simulink model "cheetahSim4trajOpt"  (R2020b)
settings: Solver=ode45  StartTime=0.0  StopTime=simTime  FixedStep=0.001  RelTol=1e-3
values from neighbouring files (symbols this model uses):
  Cd = 1.2    [cheetahTrajOpt.m]    (also in initSim.m; initSim4trajOpt.m)
  p_s = [0; 0; 0]    [cheetahEOM.m]    (also in initSim.m = [0; 0; h_b/2]; initSim4trajOpt.m = [0; 0; h_b/2])
  p_tb = p_b_com__b + [-l_b/2; 0; 0]    [cheetahEOM.m]    (also in initSim.m; initSim4trajOpt.m)
  p_tt_t = [-l_t; 0; 0]    [initSim.m]    (also in initSim4trajOpt.m)
  tau_max = 30    [cheetahTrajOpt.m]    (also in initSim4trajOpt.m)
  v = [v_x; v_y; v_z]    [cheetahEOM.m]    (also in cheetahTrajOpt.m = [10; 2; 0]; initSim.m = 0; initSim4trajOpt.m = [10; 2; 0])
  vert_b = [vert_b; vert_b - [l_b, 0, 0]]    [initSim.m]    (also in initSim4trajOpt.m)
libraries: simulink x2
settings Model: Creator=ricky  LastModifiedBy=ricky
settings SFSimCC: CustomCodeUndefinedFunction=UseInterfaceOnly

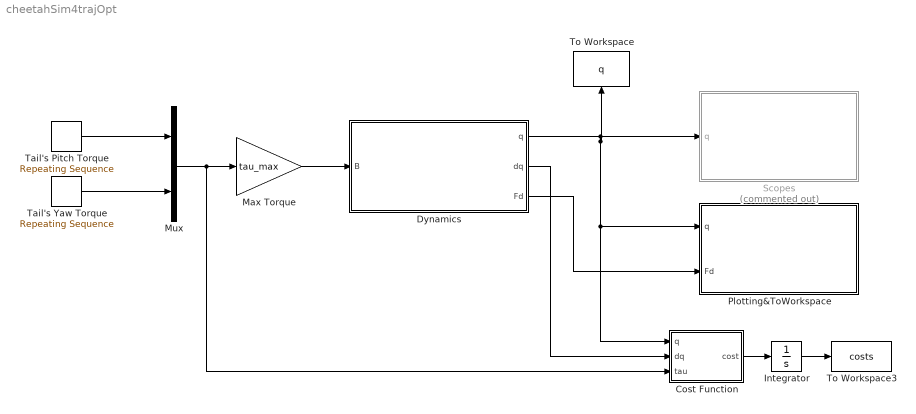
== system cheetahSim4trajOpt ==
  Cost Function : MATLAB Function  TreatAsAtomicUnit=on
  Dynamics : Subsystem
  Integrator : Integrator
  Max Torque : Gain  Gain=tau_max
  Mux : Mux  Inputs=2
  Plotting&ToWorkspace : Subsystem
  Scopes : Subsystem  Commented=on
  Tail's Pitch Torque : simulink/Sources/Repeating Sequence  rep_seq_t=timeVec  rep_seq_y=tau_th
  Tail's Yaw Torque : simulink/Sources/Repeating Sequence  rep_seq_t=timeVec  rep_seq_y=tau_psi
  To Workspace : ToWorkspace  VariableName=q  SampleTime=0.001
  To Workspace3 : ToWorkspace  VariableName=costs  SampleTime=0.001
  wires:
  Dynamics/1(q) -> Cost Function/1(q), Plotting&ToWorkspace/1(q), To Workspace/1, Scopes/1(q)
  Tail's Pitch Torque/1 -> Mux/1
  Tail's Yaw Torque/1 -> Mux/2
  Mux/1 -> Cost Function/3(tau), Max Torque/1
  Max Torque/1 -> Dynamics/1(B)
  Cost Function/1(cost) -> Integrator/1
  Integrator/1 -> To Workspace3/1
  Dynamics/3(Fd) -> Plotting&ToWorkspace/2(Fd)
  Dynamics/2(dq) -> Cost Function/2(dq)

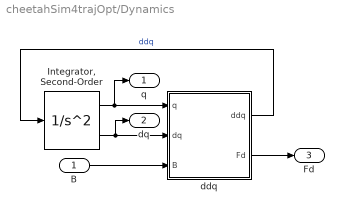
== system cheetahSim4trajOpt/Dynamics ==
  B : Inport
  "Integrator, Second-Order" : SecondOrderIntegrator  ICX=q0  ICDXDT=dq0
  ddq : MATLAB Function  TreatAsAtomicUnit=on
  q : Outport
  dq : Outport  Port=2
  Fd : Outport  Port=3
  wires:
  ddq/1(ddq) -> "Integrator, Second-Order"/1  "ddq"
  "Integrator, Second-Order"/2 -> dq/1, ddq/2(dq)
  "Integrator, Second-Order"/1 -> ddq/1(q), q/1
  B/1 -> ddq/3(B)
  ddq/2(Fd) -> Fd/1

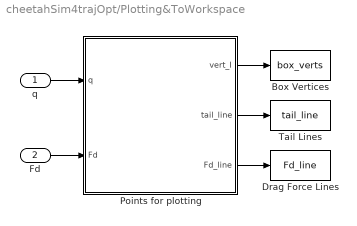
== system cheetahSim4trajOpt/Plotting&ToWorkspace ==
  q : Inport
  Fd : Inport  Port=2
  Box Vertices : ToWorkspace  VariableName=box_verts  SampleTime=-1
  Drag Force Lines : ToWorkspace  VariableName=Fd_line  SampleTime=-1
  Points for plotting : MATLAB Function  TreatAsAtomicUnit=on
  "Tail Lines " : ToWorkspace  VariableName=tail_line  SampleTime=-1
  wires:
  Fd/1 -> Points for plotting/2(Fd)
  Points for plotting/1(vert_I) -> Box Vertices/1
  Points for plotting/2(tail_line) -> "Tail Lines "/1
  q/1 -> Points for plotting/1(q)
  Points for plotting/3(Fd_line) -> Drag Force Lines/1

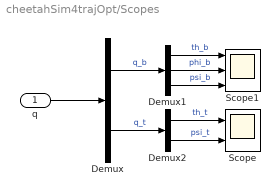
== system cheetahSim4trajOpt/Scopes ==
  q : Inport
  Demux : Demux  Outputs=2
  Demux1 : Demux  Outputs=3
  Demux2 : Demux  Outputs=2
  Scope : Scope  NumInputPorts=2
  Scope1 : Scope  NumInputPorts=3
  wires:
  Demux1/1 -> Scope1/1  "th_b"
  Demux/1 -> Demux1/1  "q_b"
  Demux2/1 -> Scope/1  "th_t"
  q/1 -> Demux/1
  Demux2/2 -> Scope/2  "psi_t"
  Demux1/2 -> Scope1/2  "phi_b"
  Demux1/3 -> Scope1/3  "psi_b"
  Demux/2 -> Demux2/1  "q_t"

== matlab function cheetahSim4trajOpt/Cost Function ==
  data: q input; dq input; tau input; cost output
function cost = cost(q, dq, tau)
    q_b = q(2:3);
    dq_b = dq(2:3);
    
    alpha = 0.5;
    cost = alpha*(q_b'*q_b + dq_b'*dq_b) + (1-alpha)*tau'*tau;
end

== matlab function cheetahSim4trajOpt/Plotting&ToWorkspace/Points for plotting ==
  data: q input; Fd input; vert_I output; tail_line output; p_s parameter; vert_b parameter; p_tb parameter; p_tt_t parameter; Fd_line output
function [vert_I, tail_line, Fd_line] = points4plot(q, Fd, p_s, vert_b, p_tb, p_tt_t)
    th_b  = q(1);
    phi_b = q(2);
    psi_b = q(3);
    th_t  = q(4);
    psi_t = q(5);
    
    vert_I = zeros(8,3);
    % box vertex locations
    R_I__b = RotZ(psi_b) * RotX(phi_b) * RotY(th_b);
    R_b__I = R_I__b';
    for idx = 1:8
        vert_I(idx, :) = (p_s + R_b__I * vert_b(idx, :)')';
    end
    % tail point locations
    R_t__I = (RotZ(psi_t) * RotY(th_t) * R_I__b)';
    p_tb_I = p_s + R_b__I*p_tb;
    p_tt_I = p_tb_I + R_t__I*p_tt_t;
    
    tail_line = [p_tb_I, p_tt_I];
    
    %drag force locations
    p_com_t = p_tt_t/2;
    p_com_I = p_tb_I + R_t__I * p_com_t;
    Fd_I = R_t__I * Fd/25; % drag forces scaled
    Fd_line = [p_com_I, Fd_I];
end
function rot = RotX(th)
    rot = [[1     0       0   ]
           [0  cos(th) sin(th)]
           [0 -sin(th) cos(th)]];
end
% function rot = RotY(th) % standard rotation about y
%     rot = [[ cos(th) 0 sin(th)]
%            [    0    1    0   ]
%            [-sin(th) 0 cos(th)]];
% end
function rot = RotY(th) % Liam's rotation about y
    rot = [[ cos(th) 0 -sin(th)]
           [    0    1    0   ]
           [sin(th) 0 cos(th)]];
end
function rot = RotZ(th)
    rot = [[ cos(th) sin(th) 0]
           [-sin(th) cos(th) 0]
           [    0       0    1]];
end

== matlab function cheetahSim4trajOpt/Dynamics/ddq ==
  data: q input size=5; ddq output size=5; dq input size=5; Cd parameter size=1; v parameter size=[3, 1]; B input size=2; Fd output
function [ddq, Fd]  = ddq( q, dq, Cd, v, B)
    coder.extrinsic('MCQ');
    coder.extrinsic('Fdrag');
    B = [0 0; 0 0; 0 0; 1 0; 0 1]*B;
    
    Fd = [0; 0; 0];
    Fd = Fdrag(q, dq, Cd, v);
    
    M = zeros(5, 5);
    C = zeros(5, 1);
    Q = zeros(5, 1);
    [M, C, Q] = MCQ(q, dq, Fd);
%     lambda = -(A*(M\A'))\(A*(M\(B-C)));
%     ddq = M\(B + Q + A'*lambda - C);
    ddq = M\(B + Q - C);
end
